simulink model "complementaryFilter"  (R2016b)
settings: Solver=VariableStepAuto  StartTime=0.0  StopTime=50  RelTol=1e-3
model workspace (MAT data in the model file):
  alpha = 0.964986376022
undefined symbols (not defined in the file): DiscIntNeverNeededParam
libraries: libEularAngleCalculator x1, simulink_extras x1
settings Model: Creator=vibek  LastModifiedBy=vibek

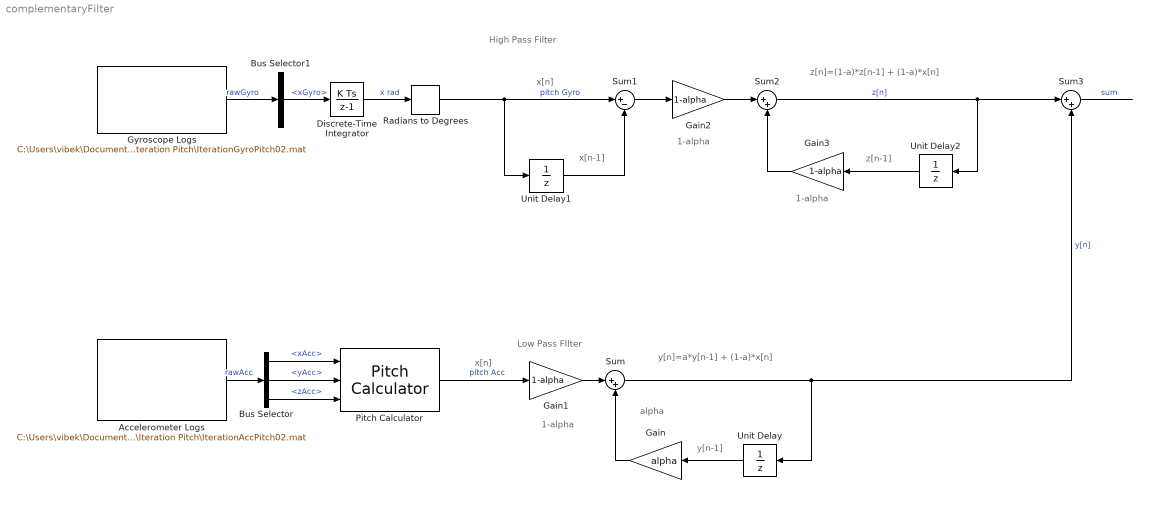
== system complementaryFilter ==
  note: High Pass Filter
  note: y[n]=a*y[n-1] + (1-a)*x[n]
  note: Low Pass FIlter
  note: x[n]
  note: x[n]
  note: x[n-1]
  note: y[n-1]
  note: 1-alpha
  note: 1-alpha
  note: alpha
  note: 1-alpha
  note: z[n]=(1-a)*z[n-1] + (1-a)*x[n]
  note: z[n-1]
  Accelerometer Logs : FromFile  FileName=C:\Users\vibek\Documents\MATLAB\Simulink\05.30.Tue\Iteration Pitch\IterationAccPitch02.mat  OutDataTypeStr=Bus: resultAcc01  SampleTime=0.01
  Bus Selector : BusSelector  OutputSignals=xAcc,yAcc,zAcc
  Bus Selector1 : BusSelector  OutputSignals=xGyro
  Discrete-Time Integrator : DiscreteIntegrator  gainval=1  InitialConditionSetting=State (most efficient)  SampleTime=-1  ICPrevOutput=DiscIntNeverNeededParam  ICPrevScaledInput=DiscIntNeverNeededParam
  Gain : Gain  Gain=alpha
  Gain1 : Gain  Gain=1-alpha
  Gain2 : Gain  Gain=1-alpha
  Gain3 : Gain  Gain=1-alpha
  Gyroscope Logs : FromFile  FileName=C:\Users\vibek\Documents\MATLAB\Simulink\05.30.Tue\Iteration Pitch\IterationGyroPitch02.mat  OutDataTypeStr=Bus: resultGyro01  SampleTime=0.01
  Pitch Calculator : libEularAngleCalculator/Pitch Calculator  Description=takes 3 inputs from accelerometer and outputs pitch value
  Radians to Degrees : simulink_extras/Transformations/Radians to Degrees
  Sum : Sum  Inputs=|++
  Sum1 : Sum  Inputs=|+-
  Sum2 : Sum  Inputs=|++
  Sum3 : Sum  Inputs=|++
  Unit Delay : UnitDelay  SampleTime=-1
  Unit Delay1 : UnitDelay  SampleTime=-1
  Unit Delay2 : UnitDelay  SampleTime=-1
  wires:
  Accelerometer Logs/1 -> Bus Selector/1  "rawAcc"
  Bus Selector/1 -> Pitch Calculator/1  "<xAcc>"
  Bus Selector/2 -> Pitch Calculator/2  "<yAcc>"
  Bus Selector/3 -> Pitch Calculator/3  "<zAcc>"
  Gyroscope Logs/1 -> Bus Selector1/1  "rawGyro"
  Bus Selector1/1 -> Discrete-Time Integrator/1  "<xGyro>"
  Discrete-Time Integrator/1 -> Radians to Degrees/1  "x rad"
  Pitch Calculator/1 -> Gain1/1  "pitch Acc"
  Radians to Degrees/1 -> Sum1/1, Unit Delay1/1  "pitch Gyro"
  Unit Delay/1 -> Gain/1
  Gain1/1 -> Sum/1
  Gain/1 -> Sum/2
  Sum/1 -> Sum3/2, Unit Delay/1  "y[n]"
  Unit Delay1/1 -> Sum1/2
  Sum1/1 -> Gain2/1
  Gain2/1 -> Sum2/1
  Sum2/1 -> Sum3/1, Unit Delay2/1  "z[n]"
  Unit Delay2/1 -> Gain3/1
  Gain3/1 -> Sum2/2
  Sum3/1 -> ?  "sum"
